simulink model "Lab_1_e1"  (R2018a)
settings: Solver=ode45  StartTime=0.0  StopTime=10  RelTol=1e-3
settings Model: Creator=WIN  LastModifiedBy=WIN

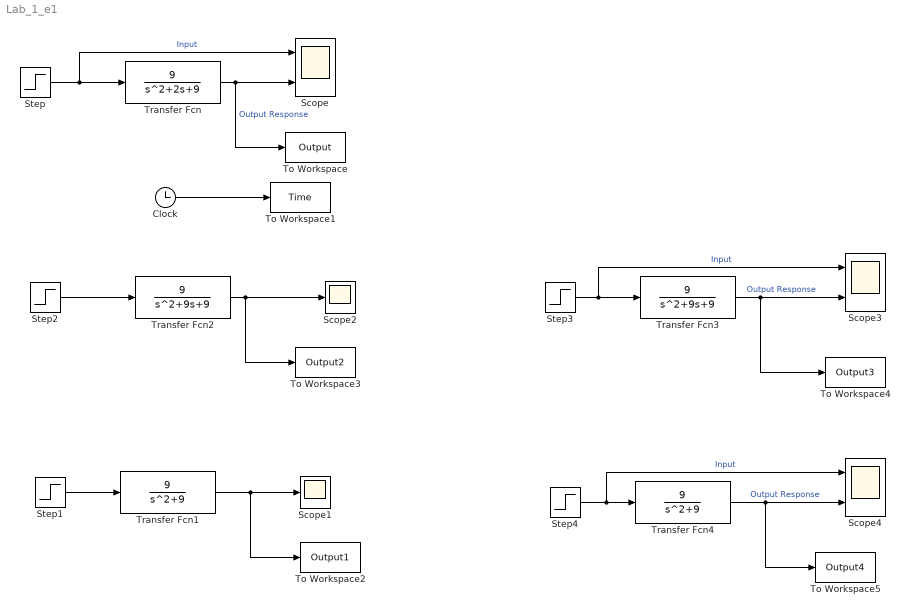
== system Lab_1_e1 ==
  Clock : Clock
  Scope : Scope  NumInputPorts=2
  Scope1 : Scope
  Scope2 : Scope
  Scope3 : Scope  NumInputPorts=2
  Scope4 : Scope  NumInputPorts=2
  Step{,1..4} (5 alike) : Step  SampleTime=0
  To Workspace : ToWorkspace  VariableName=Output  SampleTime=-1
  To Workspace1 : ToWorkspace  VariableName=Time  SampleTime=-1
  To Workspace2 : ToWorkspace  VariableName=Output1  SampleTime=-1
  To Workspace3 : ToWorkspace  VariableName=Output2  SampleTime=-1
  To Workspace4 : ToWorkspace  VariableName=Output3  SampleTime=-1
  To Workspace5 : ToWorkspace  VariableName=Output4  SampleTime=-1
  Transfer Fcn : TransferFcn  Numerator=[9]  Denominator=[1 2 9]
  Transfer Fcn1 : TransferFcn  Numerator=[9]  Denominator=[1 0 9]
  Transfer Fcn2 : TransferFcn  Numerator=[9]  Denominator=[1 9 9]
  Transfer Fcn3 : TransferFcn  Numerator=[9]  Denominator=[1 9 9]
  Transfer Fcn4 : TransferFcn  Numerator=[9]  Denominator=[1 0 9]
  wires:
  Step/1 -> Scope/1, Transfer Fcn/1  "Input"
  Transfer Fcn/1 -> Scope/2, To Workspace/1  "Output Response"
  Clock/1 -> To Workspace1/1
  Transfer Fcn1/1 -> Scope1/1, To Workspace2/1
  Step1/1 -> Transfer Fcn1/1
  Step2/1 -> Transfer Fcn2/1
  Transfer Fcn2/1 -> Scope2/1, To Workspace3/1
  Transfer Fcn3/1 -> Scope3/2, To Workspace4/1  "Output Response"
  Step3/1 -> Scope3/1, Transfer Fcn3/1  "Input"
  Step4/1 -> Scope4/1, Transfer Fcn4/1  "Input"
  Transfer Fcn4/1 -> Scope4/2, To Workspace5/1  "Output Response"
